simulink model "control_robot"  (R2020a)
settings: Solver=FixedStepAuto  StartTime=0.0  StopTime=inf  FixedStep=0.01  RelTol=1e-3
values from neighbouring files (symbols this model uses):
  alfa = 30*((2*pi)/360)    (= 0.523598775598)    [param.m]
  g = 9.8    [param.m]
  goalLoc = [2 8]    [param.m]
  L = 0.46    [param.m]
  M = 90    [param.m]
  n = 16    [param.m]
  r = 0.125    [param.m]
  simpleMap = [1 1 1 1 1 1 1 1 1 1 1 1 ... (702 elements, 26x27)]    [vid_map.mat]
  startLoc = [2 2]    [param.m]
undefined symbols (not defined in the file or in its folder): DiscIntNeverNeededParam, k_tac, motorIp, motorSp, Pot, sigbuilder_block
libraries: simulink x10, mobileRoboticsTrainingLib x8, robotalgslib x3, commchan3 x2, robotmobilelib x2, robotcorelib x2
settings Model: PacingRate=0.320000  Creator=maxim  LastModifiedBy=maxim

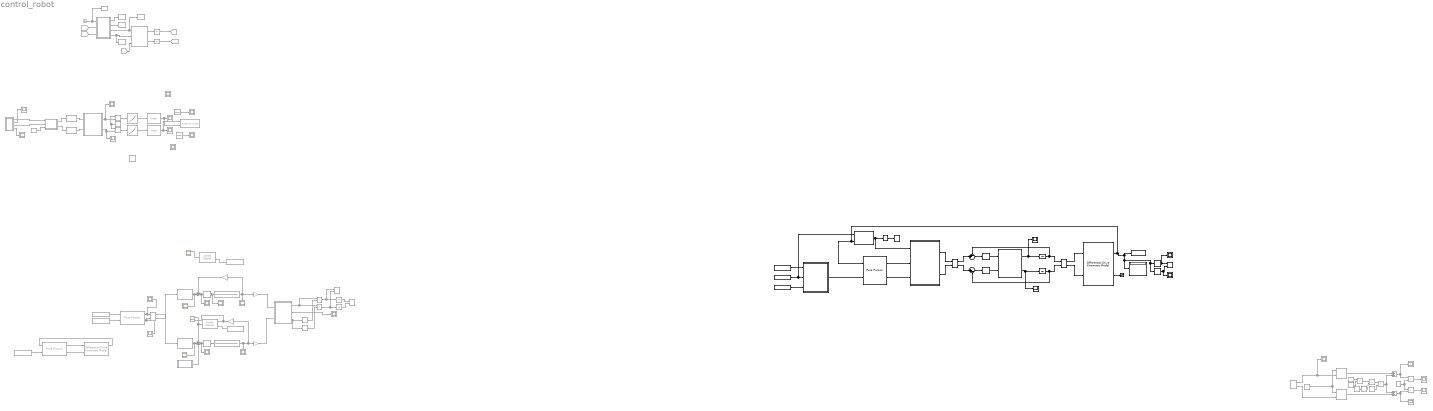
== system control_robot ==
  note: relacion de
      | transmision
  note: Volt_mot = Ktac.Vel_mot
  note: Volt_mot = Ktac.Vel_mot
  note: Voltaje salida
      | motor
  note: rad/s
  note: relacion de
      | transmision
  note: Voltaje salida
      | motor
  note: rad/s
  note: w motor derecho
  note: w motor izquierdo
  note: Robot
  note: Control de Posición
  note: Planificador de Trayectoria
  note: w/T
  note: Control Dinámco
  1-D Lookup Table1 : Lookup_n-D  Commented=on  NumberOfTableDimensions=1  BreakpointsForDimension1=motorSp  Table=motorIp  ExtrapMethod=Clip  InternalRulePriority=Speed  RndMeth=Simplest  InputSameDT=on
  1-D Lookup Table4 : Lookup_n-D  Commented=on  NumberOfTableDimensions=1  BreakpointsForDimension1=motorSp  Table=motorIp  ExtrapMethod=Clip  InternalRulePriority=Speed  RndMeth=Simplest  InputSameDT=on
  AWGN Channel : commchan3/AWGN Channel  Commented=on  InputProcessing=Columns as channels (frame based)  seed=67  noiseMode=Variance from port  EbNodB=10  EsNodB=10  SNRdB=10  bitsPerSym=1  Ps=1  Tsym=1  variance=1
  AWGN Channel1 : commchan3/AWGN Channel  Commented=on  InputProcessing=Columns as channels (frame based)  seed=67  noiseMode=Variance from port  EbNodB=10  EsNodB=10  SNRdB=10  bitsPerSym=1  Ps=1  Tsym=1  variance=1
  Add : Sum  Commented=on
  Add1 : Sum  Commented=on
  Check Distance To Goal : Subsystem
  Cinematica robot diferencial : Subsystem  Commented=on
  Cinematica Inv : robotalgslib/Pure Pursuit  DesiredLinearVelocity=3  MaxAngularVelocity=20  LookaheadDistance=0.5  TargetDirPort=off  SimulateUsing=Code generation
  Cinematica Inversa : Subsystem  Commented=on
  Clock : Clock  Commented=on
      settings: Decimation=40
  Constant : Constant  Commented=on  Value=45
  Constant1 : Constant  Commented=on  Value=Pot
  Constant10 : Constant  Commented=on  Value=alfa
  Constant11 : Constant  Commented=on  Value=r/2
  Constant12 : Constant  Commented=on  Value=1.3
  Constant2 : Constant  Commented=on  Value=[0,0; 5,0; 5,3; 0,3]  VectorParams1D=off  SampleTime=20
  Constant3 : Constant  Commented=on  Value=1570
  Constant4 : Constant  Commented=on  Value=M
  Constant5 : Constant  Commented=on  Value=0.0003  SampleTime=20
  Constant6 : Constant  Commented=on  Value=0.017  SampleTime=20
  Constant7 : Constant  Commented=on  Value=[0,0; 5,0; 5,3; 0,3]  VectorParams1D=off  SampleTime=20
  Constant8 : Constant  Commented=on  Value=[ 0, 0, 0]  SampleTime=20
  Constant9 : Constant  Commented=on  Value=g
  Differential Drive Kinematic Model : robotmobilelib/Differential Drive Kinematic Model  Commented=on  VehicleInputs=Vehicle Speed & Heading Angular Velocity  WheelRadius=r  WheelSpeedRange=[-0.6 0.6]  TrackWidth=0.2  InitialState=[0; 0; 0]  SimulateUsing=Interpreted execution
      settings: SourceProductBaseCode=RO
  Differential Drive Kinematic Model1 : robotmobilelib/Differential Drive Kinematic Model  VehicleInputs=Vehicle Speed & Heading Angular Velocity  WheelRadius=0.05  WheelSpeedRange=[-inf inf]  TrackWidth=0.2  InitialState=[startLoc, 0]'  SimulateUsing=Interpreted execution
      settings: SourceProductBaseCode=RO
  Dinamica Inversa : Subsystem
  Dinamica Inversa2 : Subsystem  Commented=on
  Discrete Derivative : simulink/Discrete/Discrete Derivative  Commented=on  gainval=1.0  ICPrevScaledInput=0.0  OutMin=[]  OutMax=[]  OutDataType=fixdt(1, 16)  OutScaling=2^-10  DoSatur=off
  Discrete Derivative1 : simulink/Discrete/Discrete Derivative  Commented=on  gainval=1.0  ICPrevScaledInput=0.0  OutMin=[]  OutMax=[]  OutDataType=fixdt(1, 16)  OutScaling=2^-10  DoSatur=off
  Discrete-Time Integrator : DiscreteIntegrator  Commented=on  SampleTime=-1  ICPrevOutput=DiscIntNeverNeededParam  ICPrevScaledInput=DiscIntNeverNeededParam
  Discrete-Time Integrator1 : DiscreteIntegrator  Commented=on  SampleTime=-1  ICPrevOutput=DiscIntNeverNeededParam  ICPrevScaledInput=DiscIntNeverNeededParam
  Display : Display
  Divide{,1..3} (4 alike) : Product  Commented=on  Inputs=*/
  From : From  Commented=on  GotoTag=P0
  From1 : From  Commented=on  GotoTag=gamma
  From2 : From  Commented=on  GotoTag=gamma
  Gain1 : Gain  Commented=on  Gain=1/n
  Gain2 : Gain  Commented=on  Gain=k_tac
  Gain4 : Gain  Commented=on  Gain=k_tac
  Gain5 : Gain  Commented=on  Gain=1/n
  Goal Location : Constant  Value=goalLoc
  Goto : Goto  Commented=on  GotoTag=gamma
  Goto1 : Goto  Commented=on  GotoTag=P0
  Integrator : Integrator  Commented=on  InitialCondition=[0;0]
  Integrator1 : Integrator  Commented=on  InitialCondition=[0;0]
  Integrator2 : Integrator  Commented=on
  Integrator3 : Integrator  Commented=on
  MATLAB Function : MATLAB Function  Commented=on  TreatAsAtomicUnit=on
  MATLAB Function1 : MATLAB Function  Commented=on  TreatAsAtomicUnit=on
  Map : Constant  Value=simpleMap
  Motor : mobileRoboticsTrainingLib/Motor  Commented=on  motorPlant=1  sensorType=Position
      settings: SourceProductName=Mobile Robotics Training Library
  Motor Der : TransferFcn  Denominator=[1]
  Motor Izq : TransferFcn  Denominator=[1]
  Motor1 : mobileRoboticsTrainingLib/Motor  Commented=on  motorPlant=1  sensorType=Position
      settings: SourceProductName=Mobile Robotics Training Library
  NOT : Logic  Operator=NOT  IconShape=distinctive  AllPortsSameDT=off  OutDataTypeStr=boolean
  PID Controller : simulink/Continuous/PID Controller  Commented=on  Controller=PID  Form=Parallel  TimeDomain=Discrete-time  UseExternalTs=off  SampleTime=-1  IntegratorMethod=Forward Euler  FilterMethod=Forward Euler  ControllerParametersSource=internal  P=1  I=1  D=0  UseFilter=on  N=100  TunerSelectOption=Transfer Function Based (PID Tuner App)  InitialConditionSource=internal  InitialConditionForIntegrator=0  InitialConditionForFilter=0  DifferentiatorICPrevScaledInput=0  ExternalReset=none  TrackingMode=off  Kt=1  LimitOutput=off  UpperSaturationLimit=inf  LowerSaturationLimit=-inf  LinearizeAsGain=on  AntiWindupMode=none  Kb=1  POutMin=[]  POutMax=[]  IOutMin=[]  IOutMax=[]  DOutMin=[]  DOutMax=[]  NOutMin=[]  NOutMax=[]  SumOutMin=[]  SumOutMax=[]  SaturationOutMin=[]  SaturationOutMax=[]  PParamMin=[]  PParamMax=[]  IParamMin=[]  IParamMax=[]  DParamMin=[]  DParamMax=[]  NParamMin=[]  NParamMax=[]  KbParamMin=[]  KbParamMax=[]  KtParamMin=[]  KtParamMax=[]  KbOutMin=[]  KbOutMax=[]  KtOutMin=[]  KtOutMax=[]  IntegratorOutMin=[]  IntegratorOutMax=[]  FilterOutMin=[]  FilterOutMax=[]  SumI1OutMin=[]  SumI1OutMax=[]  SumI2OutMin=[]  SumI2OutMax=[]  SumI3OutMin=[]  SumI3OutMax=[]  SumI4OutMin=[]  SumI4OutMax=[]  SumDOutMin=[]  SumDOutMax=[]  DifferentiatorOutMin=[]  DifferentiatorOutMax=[]  FilterDiffOutCoefMin=[]  FilterDiffOutCoefMax=[]  ReciprocalOutMin=[]  ReciprocalOutMax=[]  SumDenOutMin=[]  SumDenOutMax=[]  SumNumOutMin=[]  SumNumOutMax=[]  DivideOutMin=[]  DivideOutMax=[]  UdiffTsProdOutMin=[]  UdiffTsProdOutMax=[]  NTsProdOutMin=[]  NTsProdOutMax=[]  UintegralTsProdOutMin=[]  UintegralTsProdOutMax=[]  UngainTsProdOutMin=[]  UngainTsProdOutMax=[]  IntegratorContinuousStateAttributes=''  IntegratorStateMustResolveToSignalObject=off  IntegratorRTWStateStorageClass=Auto  FilterContinuousStateAttributes=''  FilterStateMustResolveToSignalObject=off  FilterRTWStateStorageClass=Auto  ParallelPVariant=InternalParameters  IdealPVariant=Disabled  IVariant=InternalParameters  DVariant=InternalParameters  IntegratorVariant=Discrete  SatVariant=Disabled  AWVariant=Passthrough  PCopyVariant=Disabled  TRVariant=Disabled  FdbkBlocksVariant=Forward  IdealPFdbkVariant=Disabled  SatFdbkVariant=Disabled  DerivativeFilterVariant=ForwardEulerFilter  NVariant=InternalParameters  NCopyVariant=Disabled  FilterICVariant=InternalICsFilter  IntegratorICVariant=InternalICs  ExternalResetVariant=Disabled  TRSumVariant=Passthrough  SumFdbkVariant=Disabled  SumVariant=Sum_PID  TsampFilterVariant=InternalTs  TsampNgainVariant=Passthrough  TsampIntegralVariant=Passthrough  InitialConditionSetting=Output
  PID Controller1 : simulink/Continuous/PID Controller  Commented=on  Controller=PID  Form=Parallel  TimeDomain=Continuous-time  UseExternalTs=off  SampleTime=-1  IntegratorMethod=Forward Euler  FilterMethod=Forward Euler  ControllerParametersSource=internal  P=1.83149033351054  I=8.8184370601147  D=0.0350582199329135  UseFilter=on  N=12.3100428241055  TunerSelectOption=Transfer Function Based (PID Tuner App)  InitialConditionSource=internal  InitialConditionForIntegrator=0  InitialConditionForFilter=0  DifferentiatorICPrevScaledInput=0  ExternalReset=none  TrackingMode=off  Kt=1  LimitOutput=off  UpperSaturationLimit=inf  LowerSaturationLimit=-inf  LinearizeAsGain=on  AntiWindupMode=none  Kb=1  POutMin=[]  POutMax=[]  IOutMin=[]  IOutMax=[]  DOutMin=[]  DOutMax=[]  NOutMin=[]  NOutMax=[]  SumOutMin=[]  SumOutMax=[]  SaturationOutMin=[]  SaturationOutMax=[]  PParamMin=[]  PParamMax=[]  IParamMin=[]  IParamMax=[]  DParamMin=[]  DParamMax=[]  NParamMin=[]  NParamMax=[]  KbParamMin=[]  KbParamMax=[]  KtParamMin=[]  KtParamMax=[]  KbOutMin=[]  KbOutMax=[]  KtOutMin=[]  KtOutMax=[]  IntegratorOutMin=[]  IntegratorOutMax=[]  FilterOutMin=[]  FilterOutMax=[]  SumI1OutMin=[]  SumI1OutMax=[]  SumI2OutMin=[]  SumI2OutMax=[]  SumI3OutMin=[]  SumI3OutMax=[]  SumI4OutMin=[]  SumI4OutMax=[]  SumDOutMin=[]  SumDOutMax=[]  DifferentiatorOutMin=[]  DifferentiatorOutMax=[]  FilterDiffOutCoefMin=[]  FilterDiffOutCoefMax=[]  ReciprocalOutMin=[]  ReciprocalOutMax=[]  SumDenOutMin=[]  SumDenOutMax=[]  SumNumOutMin=[]  SumNumOutMax=[]  DivideOutMin=[]  DivideOutMax=[]  UdiffTsProdOutMin=[]  UdiffTsProdOutMax=[]  NTsProdOutMin=[]  NTsProdOutMax=[]  UintegralTsProdOutMin=[]  UintegralTsProdOutMax=[]  UngainTsProdOutMin=[]  UngainTsProdOutMax=[]  IntegratorContinuousStateAttributes=''  IntegratorStateMustResolveToSignalObject=off  IntegratorRTWStateStorageClass=Auto  FilterContinuousStateAttributes=''  FilterStateMustResolveToSignalObject=off  FilterRTWStateStorageClass=Auto  ParallelPVariant=InternalParameters  IdealPVariant=Disabled  IVariant=InternalParameters  DVariant=InternalParameters  IntegratorVariant=Continuous  SatVariant=Disabled  AWVariant=Passthrough  PCopyVariant=Disabled  TRVariant=Disabled  FdbkBlocksVariant=Forward  IdealPFdbkVariant=Disabled  SatFdbkVariant=Disabled  DerivativeFilterVariant=ContFilter  NVariant=InternalParameters  NCopyVariant=Disabled  FilterICVariant=InternalICsFilter  IntegratorICVariant=InternalICs  ExternalResetVariant=Disabled  TRSumVariant=Passthrough  SumFdbkVariant=Disabled  SumVariant=Sum_PID  TsampFilterVariant=InternalTs  TsampNgainVariant=Passthrough  TsampIntegralVariant=Passthrough
  PID Controller2 : simulink/Continuous/PID Controller  Commented=on  Controller=PID  Form=Parallel  TimeDomain=Continuous-time  UseExternalTs=off  SampleTime=-1  IntegratorMethod=Forward Euler  FilterMethod=Forward Euler  ControllerParametersSource=internal  P=1.83149033351054  I=8.8184370601147  D=0.0350582199329135  UseFilter=on  N=12.3100428241055  TunerSelectOption=Transfer Function Based (PID Tuner App)  InitialConditionSource=internal  InitialConditionForIntegrator=0  InitialConditionForFilter=0  DifferentiatorICPrevScaledInput=0  ExternalReset=none  TrackingMode=off  Kt=1  LimitOutput=off  UpperSaturationLimit=inf  LowerSaturationLimit=-inf  LinearizeAsGain=on  AntiWindupMode=none  Kb=1  POutMin=[]  POutMax=[]  IOutMin=[]  IOutMax=[]  DOutMin=[]  DOutMax=[]  NOutMin=[]  NOutMax=[]  SumOutMin=[]  SumOutMax=[]  SaturationOutMin=[]  SaturationOutMax=[]  PParamMin=[]  PParamMax=[]  IParamMin=[]  IParamMax=[]  DParamMin=[]  DParamMax=[]  NParamMin=[]  NParamMax=[]  KbParamMin=[]  KbParamMax=[]  KtParamMin=[]  KtParamMax=[]  KbOutMin=[]  KbOutMax=[]  KtOutMin=[]  KtOutMax=[]  IntegratorOutMin=[]  IntegratorOutMax=[]  FilterOutMin=[]  FilterOutMax=[]  SumI1OutMin=[]  SumI1OutMax=[]  SumI2OutMin=[]  SumI2OutMax=[]  SumI3OutMin=[]  SumI3OutMax=[]  SumI4OutMin=[]  SumI4OutMax=[]  SumDOutMin=[]  SumDOutMax=[]  DifferentiatorOutMin=[]  DifferentiatorOutMax=[]  FilterDiffOutCoefMin=[]  FilterDiffOutCoefMax=[]  ReciprocalOutMin=[]  ReciprocalOutMax=[]  SumDenOutMin=[]  SumDenOutMax=[]  SumNumOutMin=[]  SumNumOutMax=[]  DivideOutMin=[]  DivideOutMax=[]  UdiffTsProdOutMin=[]  UdiffTsProdOutMax=[]  NTsProdOutMin=[]  NTsProdOutMax=[]  UintegralTsProdOutMin=[]  UintegralTsProdOutMax=[]  UngainTsProdOutMin=[]  UngainTsProdOutMax=[]  IntegratorContinuousStateAttributes=''  IntegratorStateMustResolveToSignalObject=off  IntegratorRTWStateStorageClass=Auto  FilterContinuousStateAttributes=''  FilterStateMustResolveToSignalObject=off  FilterRTWStateStorageClass=Auto  ParallelPVariant=InternalParameters  IdealPVariant=Disabled  IVariant=InternalParameters  DVariant=InternalParameters  IntegratorVariant=Continuous  SatVariant=Disabled  AWVariant=Passthrough  PCopyVariant=Disabled  TRVariant=Disabled  FdbkBlocksVariant=Forward  IdealPFdbkVariant=Disabled  SatFdbkVariant=Disabled  DerivativeFilterVariant=ContFilter  NVariant=InternalParameters  NCopyVariant=Disabled  FilterICVariant=InternalICsFilter  IntegratorICVariant=InternalICs  ExternalResetVariant=Disabled  TRSumVariant=Passthrough  SumFdbkVariant=Disabled  SumVariant=Sum_PID  TsampFilterVariant=InternalTs  TsampNgainVariant=Passthrough  TsampIntegralVariant=Passthrough
  PID Controller3 : simulink/Continuous/PID Controller  Controller=PID  Form=Parallel  TimeDomain=Continuous-time  UseExternalTs=off  SampleTime=-1  IntegratorMethod=Forward Euler  FilterMethod=Forward Euler  ControllerParametersSource=internal  P=0  I=0  D=0  UseFilter=on  N=100  TunerSelectOption=Transfer Function Based (PID Tuner App)  InitialConditionSource=internal  InitialConditionForIntegrator=0  InitialConditionForFilter=0  DifferentiatorICPrevScaledInput=0  ExternalReset=none  TrackingMode=off  Kt=1  LimitOutput=off  UpperSaturationLimit=inf  LowerSaturationLimit=-inf  LinearizeAsGain=on  AntiWindupMode=none  Kb=1  POutMin=[]  POutMax=[]  IOutMin=[]  IOutMax=[]  DOutMin=[]  DOutMax=[]  NOutMin=[]  NOutMax=[]  SumOutMin=[]  SumOutMax=[]  SaturationOutMin=[]  SaturationOutMax=[]  PParamMin=[]  PParamMax=[]  IParamMin=[]  IParamMax=[]  DParamMin=[]  DParamMax=[]  NParamMin=[]  NParamMax=[]  KbParamMin=[]  KbParamMax=[]  KtParamMin=[]  KtParamMax=[]  KbOutMin=[]  KbOutMax=[]  KtOutMin=[]  KtOutMax=[]  IntegratorOutMin=[]  IntegratorOutMax=[]  FilterOutMin=[]  FilterOutMax=[]  SumI1OutMin=[]  SumI1OutMax=[]  SumI2OutMin=[]  SumI2OutMax=[]  SumI3OutMin=[]  SumI3OutMax=[]  SumI4OutMin=[]  SumI4OutMax=[]  SumDOutMin=[]  SumDOutMax=[]  DifferentiatorOutMin=[]  DifferentiatorOutMax=[]  FilterDiffOutCoefMin=[]  FilterDiffOutCoefMax=[]  ReciprocalOutMin=[]  ReciprocalOutMax=[]  SumDenOutMin=[]  SumDenOutMax=[]  SumNumOutMin=[]  SumNumOutMax=[]  DivideOutMin=[]  DivideOutMax=[]  UdiffTsProdOutMin=[]  UdiffTsProdOutMax=[]  NTsProdOutMin=[]  NTsProdOutMax=[]  UintegralTsProdOutMin=[]  UintegralTsProdOutMax=[]  UngainTsProdOutMin=[]  UngainTsProdOutMax=[]  IntegratorContinuousStateAttributes=''  IntegratorStateMustResolveToSignalObject=off  IntegratorRTWStateStorageClass=Auto  FilterContinuousStateAttributes=''  FilterStateMustResolveToSignalObject=off  FilterRTWStateStorageClass=Auto  ParallelPVariant=InternalParameters  IdealPVariant=Disabled  IVariant=InternalParameters  DVariant=InternalParameters  IntegratorVariant=Continuous  SatVariant=Disabled  AWVariant=Passthrough  PCopyVariant=Disabled  TRVariant=Disabled  FdbkBlocksVariant=Forward  IdealPFdbkVariant=Disabled  SatFdbkVariant=Disabled  DerivativeFilterVariant=ContFilter  NVariant=InternalParameters  NCopyVariant=Disabled  FilterICVariant=InternalICsFilter  IntegratorICVariant=InternalICs  ExternalResetVariant=Disabled  TRSumVariant=Passthrough  SumFdbkVariant=Disabled  SumVariant=Sum_PID  TsampFilterVariant=InternalTs  TsampNgainVariant=Passthrough  TsampIntegralVariant=Passthrough
  PID Controller4 : simulink/Continuous/PID Controller  Controller=PID  Form=Parallel  TimeDomain=Continuous-time  UseExternalTs=off  SampleTime=-1  IntegratorMethod=Forward Euler  FilterMethod=Forward Euler  ControllerParametersSource=internal  P=0  I=0  D=0  UseFilter=on  N=100  TunerSelectOption=Transfer Function Based (PID Tuner App)  InitialConditionSource=internal  InitialConditionForIntegrator=0  InitialConditionForFilter=0  DifferentiatorICPrevScaledInput=0  ExternalReset=none  TrackingMode=off  Kt=1  LimitOutput=off  UpperSaturationLimit=inf  LowerSaturationLimit=-inf  LinearizeAsGain=on  AntiWindupMode=none  Kb=1  POutMin=[]  POutMax=[]  IOutMin=[]  IOutMax=[]  DOutMin=[]  DOutMax=[]  NOutMin=[]  NOutMax=[]  SumOutMin=[]  SumOutMax=[]  SaturationOutMin=[]  SaturationOutMax=[]  PParamMin=[]  PParamMax=[]  IParamMin=[]  IParamMax=[]  DParamMin=[]  DParamMax=[]  NParamMin=[]  NParamMax=[]  KbParamMin=[]  KbParamMax=[]  KtParamMin=[]  KtParamMax=[]  KbOutMin=[]  KbOutMax=[]  KtOutMin=[]  KtOutMax=[]  IntegratorOutMin=[]  IntegratorOutMax=[]  FilterOutMin=[]  FilterOutMax=[]  SumI1OutMin=[]  SumI1OutMax=[]  SumI2OutMin=[]  SumI2OutMax=[]  SumI3OutMin=[]  SumI3OutMax=[]  SumI4OutMin=[]  SumI4OutMax=[]  SumDOutMin=[]  SumDOutMax=[]  DifferentiatorOutMin=[]  DifferentiatorOutMax=[]  FilterDiffOutCoefMin=[]  FilterDiffOutCoefMax=[]  ReciprocalOutMin=[]  ReciprocalOutMax=[]  SumDenOutMin=[]  SumDenOutMax=[]  SumNumOutMin=[]  SumNumOutMax=[]  DivideOutMin=[]  DivideOutMax=[]  UdiffTsProdOutMin=[]  UdiffTsProdOutMax=[]  NTsProdOutMin=[]  NTsProdOutMax=[]  UintegralTsProdOutMin=[]  UintegralTsProdOutMax=[]  UngainTsProdOutMin=[]  UngainTsProdOutMax=[]  IntegratorContinuousStateAttributes=''  IntegratorStateMustResolveToSignalObject=off  IntegratorRTWStateStorageClass=Auto  FilterContinuousStateAttributes=''  FilterStateMustResolveToSignalObject=off  FilterRTWStateStorageClass=Auto  ParallelPVariant=InternalParameters  IdealPVariant=Disabled  IVariant=InternalParameters  DVariant=InternalParameters  IntegratorVariant=Continuous  SatVariant=Disabled  AWVariant=Passthrough  PCopyVariant=Disabled  TRVariant=Disabled  FdbkBlocksVariant=Forward  IdealPFdbkVariant=Disabled  SatFdbkVariant=Disabled  DerivativeFilterVariant=ContFilter  NVariant=InternalParameters  NCopyVariant=Disabled  FilterICVariant=InternalICsFilter  IntegratorICVariant=InternalICs  ExternalResetVariant=Disabled  TRSumVariant=Passthrough  SumFdbkVariant=Disabled  SumVariant=Sum_PID  TsampFilterVariant=InternalTs  TsampNgainVariant=Passthrough  TsampIntegralVariant=Passthrough
  Planner : MATLAB Function  TreatAsAtomicUnit=on
  Product{,1..6} (7 alike) : Product  Commented=on
  Pure Pursuit : robotalgslib/Pure Pursuit  Commented=on  DesiredLinearVelocity=3  MaxAngularVelocity=20  LookaheadDistance=0.5  TargetDirPort=off  SimulateUsing=Interpreted execution
  Pure Pursuit1 : robotalgslib/Pure Pursuit  Commented=on  DesiredLinearVelocity=3  MaxAngularVelocity=20  LookaheadDistance=0.5  TargetDirPort=off  SimulateUsing=Interpreted execution
  Px vs Py : simulink/Sinks/XY Graph  Commented=on  xmin=-5  xmax=5  ymin=-5  ymax=5  st=-1
  Robot Simulator1 : mobileRoboticsTrainingLib/Robot Simulator  Priority=99  Commented=on  mapVar=[]  startX=1  startY=1  startTheta=0  axleLength=0.1  wheelR=0.05
  Scope{,1..13,15..17,19..21} (20 alike) : Scope  Commented=on
  Scope14 : Scope  Commented=on  NumInputPorts=2
  Scope18 : Scope  Commented=on  NumInputPorts=2
  Selector : Selector  InputPortWidth=3  IndexOptions=Index vector (dialog)  Indices=[1]  OutputSizes=1
  Selector1 : Selector  InputPortWidth=3  IndexOptions=Index vector (dialog)  Indices=[2]  OutputSizes=1
  Signal Builder : Subsystem  Tag=STV Subsys  Commented=on  LoadFcn=sigbuilder_block('load');  StartFcn=sigbuilder_block('start');  StopFcn=sigbuilder_block('stop');  ClipboardFcn=sigbuilder_block('clipboard');  mask(Sigbuilder block){tuvar=[0:10]}
      mask help: Simulink:masks:SigbuilderBlock_MD
      mask init:
      | if ~strcmp(get_param(bdroot(gcbh),'SimulationStatus'),'stopped') tuvar = sigbuilder_block('maskInit'); end
      settings: CopyFcn=sigbuilder_block('copy');  DeleteFcn=sigbuilder_block('delete');  ModelCloseFcn=sigbuilder_block('modelClose');  PreSaveFcn=sigbuilder_block('preSave');  PauseFcn=sigbuilder_block('pause');  ContinueFcn=sigbuilder_block('continue');  NameChangeFcn=sigbuilder_block('namechange');  OpenFcn=sigbuilder_block('open',[321 79.8 550.8 400.2 ]);  CloseFcn=sigbuilder_block('close');
      mask Display: plot(0, 0, 100, 100,[2, 2, 32, 32, 2], [68, 8, 8, 68, 68],[32, 2], [38, 38], [32, 19, 2],[53, 60, 44], [32, 17, 17, 2],[16, 16, 31, 31]);txt = getActiveGroup(gcbh);text(2, 100, txt,'verticalAlignment', 'top');
  Sin : Trigonometry  Commented=on
  Start Location : Constant  Value=startLoc
  Stop Simulation : Stop
  Sum : Sum  Commented=on  Inputs=-+|
  Sum1 : Sum  Inputs=-+|
  Sum2 : Sum  Commented=on  Inputs=-+-
  Sum3 : Sum  Inputs=|+-
  Terminator : Terminator
  To Workspace : ToWorkspace  VariableName=Pose  SampleTime=-1
  To Workspace1 : ToWorkspace  Commented=on  VariableName=v  SampleTime=-1
  To Workspace2 : ToWorkspace  Commented=on  VariableName=t  SampleTime=-1
  To Workspace3 : ToWorkspace  Commented=on  VariableName=P  SampleTime=-1
  To Workspace4 : ToWorkspace  Commented=on  VariableName=Pd  SampleTime=-1
  To Workspace5 : ToWorkspace  Commented=on  VariableName=w  SampleTime=-1
  To vw : mobileRoboticsTrainingLib/To vw  axleLength=0.1  wheelR=0.05
      settings: SourceProductName=Mobile Robotics Training Library
  To wlwr : mobileRoboticsTrainingLib/To wlwr  Commented=on  axleLength=L  wheelR=r
      link override change parameters: Gain=[1 -L/2; 1 L/2]
      link override vtow: Gain=1/r
  To wlwr1 : mobileRoboticsTrainingLib/To wlwr  axleLength=0.1  wheelR=0.05
  To wlwr3 : mobileRoboticsTrainingLib/To wlwr  Commented=on  axleLength=0.1  wheelR=0.05
  Torque Der1 : Scope  Commented=on
  Torque Der2 : Scope  Commented=on
  Torque Derecho : Scope
  Torque Izq1 : Scope  Commented=on
  Torque Izq2 : Scope  Commented=on
  Torque Izq6 : Scope  Commented=on
  Torque Izquierdo : Scope
  Trayectoria : Subsystem  Commented=on
  Trigonometric Function : Trigonometry  Commented=on
  Trigonometric Function1 : Trigonometry  Commented=on  Operator=cos
  Vx vs Vy : simulink/Sinks/XY Graph  Commented=on  xmin=-0.2  xmax=0.2  ymin=-0.2  ymax=0.2  st=-1
  XY Graph : simulink/Sinks/XY Graph  xmin=0  xmax=28  ymin=0  ymax=28  st=-1
  Zero-Velocity At Goal : Subsystem
  vel angular motor / voltaje : TransferFcn  Commented=on  Numerator=[0.112]  Denominator=[5.3e-5 0.031 0.109]
  vel angular motor / voltaje1 : TransferFcn  Commented=on  Numerator=[0.062]  Denominator=[5.3e-5 0.031 0.109]
  vel2volt : Subsystem  Commented=on
  vel2volt1 : Subsystem  Commented=on
  x : Scope
  y : Scope
  wires:
  Clock/1 -> To Workspace2/1, MATLAB Function/1(t)
  MATLAB Function/3(v) -> To Workspace1/1, MATLAB Function1/1(v)
  From1/1 -> MATLAB Function/3(gamma)
  From/1 -> MATLAB Function/2(P0)
  MATLAB Function/2(P) -> To Workspace3/1
  MATLAB Function/1(Pd) -> To Workspace4/1
  MATLAB Function/4(w) -> To Workspace5/1, MATLAB Function1/2(w)
  MATLAB Function1/1(dP0) -> Integrator/1
  MATLAB Function1/2(dgamma) -> Integrator1/1
  Integrator1/1 -> Goto/1
  Integrator/1 -> Goto1/1
  From2/1 -> MATLAB Function1/3(gamma)
  Discrete-Time Integrator/1 -> Scope2/1
  Discrete-Time Integrator1/1 -> Scope3/1
  Cinematica Inversa/2(wl) -> Discrete Derivative/1
  Discrete Derivative/1 -> Dinamica Inversa2/2(ddthetaL)
  Cinematica Inversa/1(wr) -> Discrete Derivative1/1
  Discrete Derivative1/1 -> Dinamica Inversa2/1(ddthetaR)
  Dinamica Inversa2/2(tauTot_L) -> Divide1/2, Scope5/1
  Trayectoria/1(x) -> Cinematica Inversa/1(xd)
  Trayectoria/3(y) -> Cinematica Inversa/2(yd)
  Trayectoria/2(dx) -> Scope6/1
  Trayectoria/4(dy) -> Scope7/1
  Constant/1 -> Cinematica Inversa/3(gamma)
  Dinamica Inversa2/1(tauTot_R) -> Divide/2, Scope4/1
  Constant1/1 -> Divide1/1, Divide/1
  Divide/1 -> 1-D Lookup Table4/1
  1-D Lookup Table1/1 -> Motor1/1
  1-D Lookup Table4/1 -> Motor/1
  Divide1/1 -> 1-D Lookup Table1/1
  Motor/1 -> Robot Simulator1/2, Scope8/1
  Motor1/1 -> Robot Simulator1/1, Scope9/1
  vel angular motor / voltaje/1 -> Gain2/1, Scope10/1, Gain1/1
  Gain5/1 -> Cinematica robot diferencial/2(w_l)
  Trigonometric Function/1 -> Product/2
  Constant8/1 -> Pure Pursuit/1
  PID Controller1/1 -> Scope11/1, vel angular motor / voltaje/1
  Product/1 -> Integrator2/1, Vx vs Vy/1
  Pure Pursuit/2 -> Scope21/1, To wlwr/2
  Constant6/1 -> AWGN Channel1/2
  Cinematica robot diferencial/1(v robot) -> Product/1, Product1/1
  To wlwr/2 -> vel2volt/1(vel motor)
  Cinematica robot diferencial/2(w robot) -> Scope15/1
  Integrator3/1 -> Px vs Py/2
  AWGN Channel1/1 -> Scope14/1, Sum2/1
  To wlwr/1 -> vel2volt1/1(vel motor)
  PID Controller2/1 -> vel angular motor / voltaje1/1
  Signal Builder/1(Pert) -> Sum2/3
  Trigonometric Function1/1 -> Product1/2
  Gain1/1 -> Cinematica robot diferencial/1(w_r)
  vel angular motor / voltaje1/1 -> Gain5/1, Gain4/1, Scope19/1
  Cinematica robot diferencial/3(theta) -> Trigonometric Function1/1, Trigonometric Function/1
  Gain4/1 -> Scope14/2, AWGN Channel1/1
  Pure Pursuit/1 -> Scope20/1, To wlwr/1
  Constant5/1 -> AWGN Channel/2
  Sum/1 -> Scope16/1, PID Controller1/1
  Constant7/1 -> Pure Pursuit/2
  Sum2/1 -> PID Controller2/1, Scope12/1
  AWGN Channel/1 -> Scope18/1
  Product1/1 -> Vx vs Vy/2, Integrator3/1
  Integrator2/1 -> Px vs Py/1
  vel2volt/1(voltaje) -> Scope17/1, Sum/2
  vel2volt1/1(voltaje) -> Sum2/2, Scope13/1
  Gain2/1 -> Sum/1
  Pure Pursuit1/1 -> Differential Drive Kinematic Model/1
  Pure Pursuit1/2 -> Differential Drive Kinematic Model/2
  Constant2/1 -> Pure Pursuit1/2
  Differential Drive Kinematic Model/1 -> Pure Pursuit1/1
  Map/1 -> Planner/3(mapMatrix)
  Differential Drive Kinematic Model1/2 -> Terminator/1
  NOT/1 -> Stop Simulation/1
  Differential Drive Kinematic Model1/1 -> To Workspace/1, Selector1/1, Selector/1, Display/1, Cinematica Inv/1, Check Distance To Goal/2(currentPose)
  Start Location/1 -> Planner/1(startPos)
  Cinematica Inv/1 -> Zero-Velocity At Goal/2(linearVelocityOutput)  "linearVelocityOutput"
  Selector1/1 -> y/1, XY Graph/2
  Check Distance To Goal/1(atGoal) -> Zero-Velocity At Goal/1(atGoal), NOT/1
  Cinematica Inv/2 -> Zero-Velocity At Goal/3(angularVelocityOutput)  "angularVelocityOutput"
  Planner/1(waypoints) -> Cinematica Inv/2  "planOutput"
  Goal Location/1 -> Check Distance To Goal/1(robotGoal), Planner/2(endPos)
  Product5/1 -> Torque Izq2/1
  Product6/1 -> Torque Der2/1
  Constant3/1 -> Divide2/1, Divide3/1
  Selector/1 -> x/1, XY Graph/1
  Constant4/1 -> Product2/1
  Constant9/1 -> Product2/2
  Product2/1 -> Product3/1
  Constant10/1 -> Sin/1
  Sin/1 -> Product3/2
  Add/1 -> Torque Izq1/1, Product5/1
  Divide2/1 -> Add/1
  Add1/1 -> Product6/2, Torque Der1/1
  Divide3/1 -> Add1/2
  Product3/1 -> Product4/1
  Constant11/1 -> Product4/2
  Product4/1 -> Add/2, Add1/1
  Constant12/1 -> Product6/1, Product5/2
  Dinamica Inversa/2(tauTot_R) -> Motor Der/1, Torque Derecho/1
  Dinamica Inversa/1(tauTot_L) -> Motor Izq/1, Torque Izquierdo/1
  To wlwr3/1 -> Torque Izq6/1, Divide2/2
  To wlwr3/2 -> Divide3/2
  Sum1/1 -> PID Controller3/1
  Sum3/1 -> PID Controller4/1
  Motor Der/1 -> To vw/2, Sum3/2
  Motor Izq/1 -> To vw/1, Sum1/1
  To vw/1 -> Differential Drive Kinematic Model1/1
  To vw/2 -> Differential Drive Kinematic Model1/2
  To wlwr1/1 -> Sum1/2
  To wlwr1/2 -> Sum3/1
  PID Controller3/1 -> Dinamica Inversa/1(ddthetaR)
  PID Controller4/1 -> Dinamica Inversa/2(ddthetaL)
  Zero-Velocity At Goal/1(Linear Velocity) -> To wlwr1/1
  Zero-Velocity At Goal/2(Angular Velocity) -> To wlwr1/2

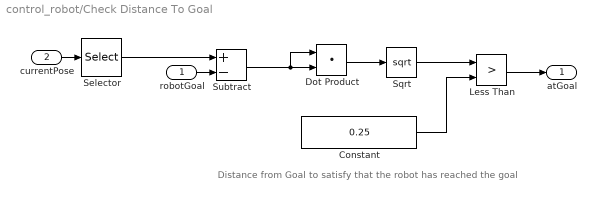
== system control_robot/Check Distance To Goal ==
  note: Distance from Goal to satisfy that the robot has reached the goal
  robotGoal : Inport
  currentPose : Inport  Port=2
  Constant : Constant  Value=0.25
  Dot Product : DotProduct  InputSameDT=on  OutDataTypeStr=Inherit: Inherit via internal rule
  Less Than : RelationalOperator  Operator=>  OutDataTypeStr=boolean  RndMeth=Simplest
  Selector : Selector  InputPortWidth=3  IndexOptions=Index vector (dialog)  Indices=[1 2]  OutputSizes=1
  Sqrt : Sqrt  SaturateOnIntegerOverflow=on
  Subtract : Sum  Inputs=+-
  atGoal : Outport
  wires:
  robotGoal/1 -> Subtract/2
  Dot Product/1 -> Sqrt/1
  Constant/1 -> Less Than/2
  currentPose/1 -> Selector/1
  Less Than/1 -> atGoal/1
  Sqrt/1 -> Less Than/1
  Subtract/1 -> Dot Product/1, Dot Product/2
  Selector/1 -> Subtract/1

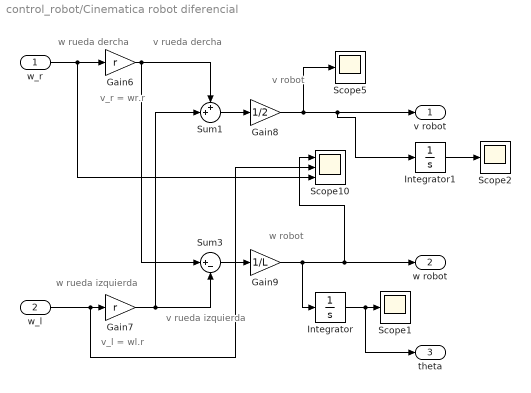
== system control_robot/Cinematica robot diferencial ==
  note: w rueda
      | dercha
  note: w rueda
      | izquierda
  note: v_r = wr.r
  note: v_l = wl.r
  note: v robot
  note: w robot
  note: v rueda
      | dercha
  note: v rueda
      | izquierda
  w_r : Inport
  w_l : Inport  Port=2
  Gain6 : Gain  Gain=r
  Gain7 : Gain  Gain=r
  Gain8 : Gain  Gain=1/2
  Gain9 : Gain  Gain=1/L
  Integrator : Integrator
  Integrator1 : Integrator
  Scope1 : Scope
  Scope10 : Scope  NumInputPorts=3
  Scope2 : Scope
  Scope5 : Scope
  Sum1 : Sum  Inputs=++|
  Sum3 : Sum  Inputs=|+-
  v robot : Outport
  w robot : Outport  Port=2
  theta : Outport  Port=3
  wires:
  w_l/1 -> Scope10/2, Gain7/1
  Sum3/1 -> Gain9/1
  Gain9/1 -> Integrator/1, w robot/1, Scope10/1
  Gain7/1 -> Sum3/2, Sum1/2
  Gain6/1 -> Sum3/1, Sum1/1
  Sum1/1 -> Gain8/1
  w_r/1 -> Scope10/3, Gain6/1
  Gain8/1 -> Scope5/1, Integrator1/1, v robot/1
  Integrator/1 -> theta/1, Scope1/1
  Integrator1/1 -> Scope2/1

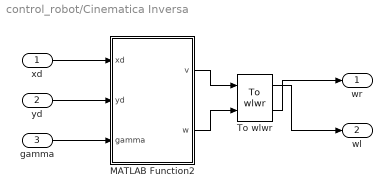
== system control_robot/Cinematica Inversa ==
  xd : Inport
  yd : Inport  Port=2
  gamma : Inport  Port=3
  MATLAB Function2 : MATLAB Function  TreatAsAtomicUnit=on
  To wlwr : mobileRoboticsTrainingLib/To wlwr  axleLength=L  wheelR=r
      link override change parameters: Gain=[1 -L/2; 1 L/2]
      link override vtow: Gain=1/r
  wr : Outport
  wl : Outport  Port=2
  wires:
  MATLAB Function2/2(w) -> To wlwr/2
  MATLAB Function2/1(v) -> To wlwr/1
  gamma/1 -> MATLAB Function2/3(gamma)
  yd/1 -> MATLAB Function2/2(yd)
  xd/1 -> MATLAB Function2/1(xd)
  To wlwr/2 -> wr/1
  To wlwr/1 -> wl/1

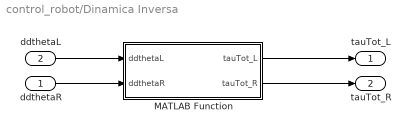
== system control_robot/Dinamica Inversa ==
  ddthetaR : Inport
  ddthetaL : Inport  Port=2
  MATLAB Function : MATLAB Function  TreatAsAtomicUnit=on
  tauTot_L : Outport
  tauTot_R : Outport  Port=2
  wires:
  ddthetaL/1 -> MATLAB Function/1(ddthetaL)
  ddthetaR/1 -> MATLAB Function/2(ddthetaR)
  MATLAB Function/2(tauTot_R) -> tauTot_R/1
  MATLAB Function/1(tauTot_L) -> tauTot_L/1

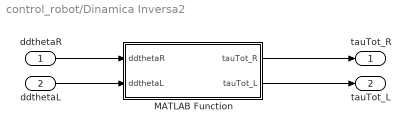
== system control_robot/Dinamica Inversa2 ==
  ddthetaR : Inport
  ddthetaL : Inport  Port=2
  MATLAB Function : MATLAB Function  TreatAsAtomicUnit=on
  tauTot_R : Outport
  tauTot_L : Outport  Port=2
  wires:
  ddthetaL/1 -> MATLAB Function/2(ddthetaL)
  ddthetaR/1 -> MATLAB Function/1(ddthetaR)
  MATLAB Function/1(tauTot_R) -> tauTot_R/1
  MATLAB Function/2(tauTot_L) -> tauTot_L/1

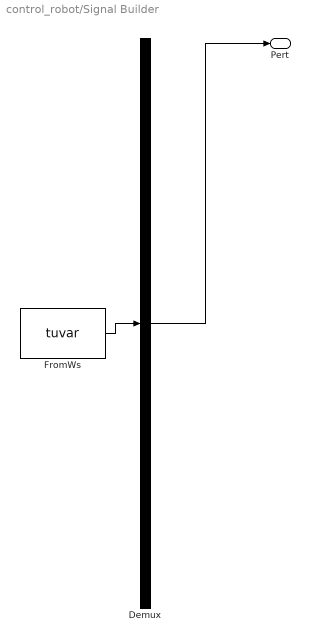
== system control_robot/Signal Builder ==
  Demux : Demux  Tag=STV Demux  Outputs=1
      settings: DisplayOption=none
  FromWs : FromWorkspace  Tag=STV FromWs  VariableName=tuvar  SampleTime=0.01
      SigBuilderData=|
      | common.afterFinalStr = 'Extrapolate'
      | common.sampleTime = '0.01'
      | dataSet.timeRange = [0 20]
      | dataSet.name = 'Group 1'
      | sbobj.Groups.Name = 'Group 1'
      | sbobj.Groups.Signals.Name = 'Pert'
      | sbobj.Groups.Signals.XData = [0 4 4 6 6 20]
      | sbobj.Groups.Signals.YData = [0 0 1 1 0 0]
      | sbobj.Groups.TimeRange = [0 20]
  Pert : Outport  Tag=STV Outport
  wires:
  Demux/1 -> Pert/1
  FromWs/1 -> Demux/1

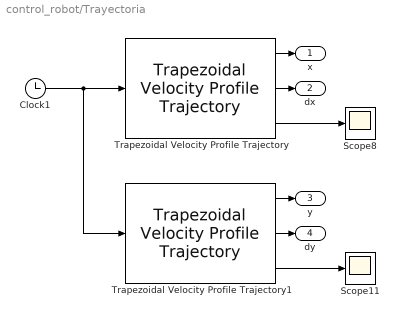
== system control_robot/Trayectoria ==
  Clock1 : Clock
  Scope11 : Scope
  Scope8 : Scope
  Trapezoidal Velocity Profile Trajectory : robotcorelib/Trapezoidal Velocity Profile Trajectory  WaypointSource=Internal  Waypoints=[ 0, -0.5, -1 ]  NumParams=0  Parameter1=Peak Velocity  Parameter2=End Time  ParameterSource=Internal  PeakVelocity=[ 2; 2 ]  Acceleration=[ 1; 2 ]  EndTime=[ 1; 1 ]  AccelTime=[ 1; 2 ]  SimulateUsing=Interpreted execution
      settings: SourceProductBaseCode=NV,RO,RR
  Trapezoidal Velocity Profile Trajectory1 : robotcorelib/Trapezoidal Velocity Profile Trajectory  WaypointSource=Internal  Waypoints=[ 0, 0.5, 1 ]  NumParams=0  Parameter1=Peak Velocity  Parameter2=End Time  ParameterSource=Internal  PeakVelocity=[ 2; 2 ]  Acceleration=[ 1; 2 ]  EndTime=[ 1; 1 ]  AccelTime=[ 1; 2 ]  SimulateUsing=Interpreted execution
      settings: SourceProductBaseCode=NV,RO,RR
  x : Outport
  dx : Outport  Port=2
  y : Outport  Port=3
  dy : Outport  Port=4
  wires:
  Trapezoidal Velocity Profile Trajectory1/3 -> Scope11/1
  Trapezoidal Velocity Profile Trajectory/3 -> Scope8/1
  Trapezoidal Velocity Profile Trajectory1/1 -> y/1
  Trapezoidal Velocity Profile Trajectory/2 -> dx/1
  Clock1/1 -> Trapezoidal Velocity Profile Trajectory1/1, Trapezoidal Velocity Profile Trajectory/1
  Trapezoidal Velocity Profile Trajectory1/2 -> dy/1
  Trapezoidal Velocity Profile Trajectory/1 -> x/1

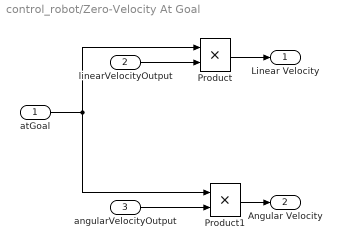
== system control_robot/Zero-Velocity At Goal ==
  atGoal : Inport
  linearVelocityOutput : Inport  Port=2
  angularVelocityOutput : Inport  Port=3
  Product : Product
  Product1 : Product
  Linear Velocity : Outport  OutDataTypeStr=double
  Angular Velocity : Outport  Port=2  OutDataTypeStr=double
  wires:
  atGoal/1 -> Product1/1, Product/1
  angularVelocityOutput/1 -> Product1/2
  linearVelocityOutput/1 -> Product/2
  Product/1 -> Linear Velocity/1
  Product1/1 -> Angular Velocity/1

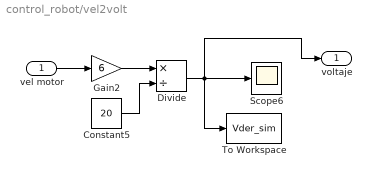
== system control_robot/vel2volt ==
  vel motor : Inport
  Constant5 : Constant  Value=20
  Divide : Product  Inputs=*/
  Gain2 : Gain  Gain=6
  Scope6 : Scope
  To Workspace : ToWorkspace  VariableName=Vder_sim  SampleTime=-1
  voltaje : Outport
  wires:
  Divide/1 -> voltaje/1, Scope6/1, To Workspace/1
  Gain2/1 -> Divide/1
  Constant5/1 -> Divide/2
  vel motor/1 -> Gain2/1

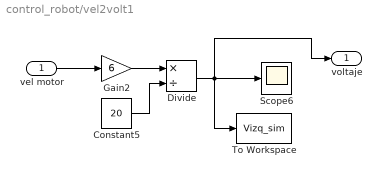
== system control_robot/vel2volt1 ==
  vel motor : Inport
  Constant5 : Constant  Value=20
  Divide : Product  Inputs=*/
  Gain2 : Gain  Gain=6
  Scope6 : Scope
  To Workspace : ToWorkspace  VariableName=Vizq_sim  SampleTime=-1
  voltaje : Outport
  wires:
  vel motor/1 -> Gain2/1
  Constant5/1 -> Divide/2
  Gain2/1 -> Divide/1
  Divide/1 -> To Workspace/1, Scope6/1, voltaje/1

== matlab function control_robot/MATLAB Function1 ==
  data: v input; w input; gamma input; dP0 output; dgamma output
function [dP0,dgamma] = SNL(v, w, gamma)
dP0 = [v*cos(gamma); v*sin(gamma)]
dgamma = w;

== matlab function control_robot/MATLAB Function ==
  data: Pd output; P output; t input; P0 input; v output; gamma input; w output
function [Pd, P, v, w] = Pout(t, P0, gamma)
%control tomando un punto por fuera
d = 0.1; kp = 2;

%trayectoria deseada
T=40;
b = 2*pi/T;
Pd = [cos(b*t); sin(b*t)];
dPd = [-b*sin(b*t); b*cos(b*t)];

%Punto por fuera del eje de las ruedas
P = [P0(1)+d*cos(gamma); P0(2)+d*sin(gamma)];

%Error de seguimiento
e = Pd-P;

%Matriz de desacoplamiento o Jacboiano
A = [cos(gamma), -d*sin(gamma);
     sin(gamma), d*cos(gamma)];

 %Control P con compensación
 u = dPd + kp*e;
 U = A\u;
 v = U(1);
 w = U(2);

== matlab function control_robot/Cinematica Inversa/MATLAB Function2 ==
  data: xd input; yd input; v output; gamma input; w output
 function [v, w] = cin_inv(xd, yd, gamma)
%control tomando un punto por fuera
a = 0.445; 

%Matriz de desacoplamiento o Jacboiano
A = [cos(gamma), -a*sin(gamma);
     sin(gamma), a*cos(gamma)]

%Control P con compensación
P = [xd; yd];
U = A^(-1)*P ;
v = U(1);
w = U(2);

== matlab function control_robot/Dinamica Inversa2/MATLAB Function ==
  data: ddthetaR input; ddthetaL input; tauTot_R output; tauTot_L output
function [tauTot_R, tauTot_L] = din_inv(ddthetaR, ddthetaL)

a = 0.445;
L = 0.46;
r = 0.125;

M = 90;
mg = 1.5;
mc = 1;
rc = 0.08;
I = 8.53;
alfa = 30;
mu = 80;
g = 9.8;


ddtheta = [ddthetaR; ddthetaL] %Vector de aceleraciones
D = (r/(L^2))*[(M*(a^2) + 1/4 + I +(M*a*L)/r + 2*(L^2)*(2*mc + mg)),  -(M*(a^2) + 1/4 - I);
                  -(M*(a^2) + 1/4 - I), (M*(a^2) + 1/4 + I -(M*a*L)/r + 2*(L^2)*(2*mc + mg))]; %Matriz de inercia

tau_ef = D * ddtheta;

tau_fric = 0.3 * tau_ef; %Torques de friccion

tau_pend = (r/2)*mu*g*sin(alfa)*[1;1]; %Torques de pendiente de 30 grados

tauTot = tau_ef + tau_fric + tau_pend;

tauTot_R = tauTot(1); 
tauTot_L = tauTot(2);

== matlab function control_robot/Planner ==
  settings: updateMethod=DISCRETE
  data: startPos input size=[1 2]; endPos input size=[1 2]; waypoints output size=[100 2]; mapMatrix input
function waypoints = planning(startPos, endPos, mapMatrix)

persistent waypointsInternal
persistent prevStartPos
persistent prevEndPos

% Set constant parameters
maxNumNodes = 100;

% Initialize persistent variables that are used downstream
if isempty(prevStartPos)
    prevStartPos = startPos;
end

if isempty(prevEndPos)
    prevEndPos = endPos;
end

isNewPath = (~isequal(prevStartPos, startPos) || ~isequal(prevEndPos, endPos));

if isempty(waypointsInternal) || isNewPath
    % Two conditions in which waypoints must be set: they are not yet
    % initialized, or they are initialized, but the current start and end
    % do not match those used to generate the previous set of waypoints
    [waypointsInternal] = planPath(mapMatrix, maxNumNodes, startPos, endPos);
end

% Update the outputs
waypoints = waypointsInternal;

% Update the persistent variables that indicate previous state
prevStartPos = startPos;
prevEndPos = endPos;

%% Helper Function

function wayPoints = planPath(mapMatrix, maxNodes, startPos, endPos)
    
    % Create a probabilistic roadmap
    map = binaryOccupancyMap(mapMatrix);
    prm = mobileRobotPRM(map, maxNodes);
    
    % Find a path between two points
    xy = findpath(prm, startPos, endPos);
    wayPoints = repmat(endPos, maxNodes, 1);
    
    % Number of nodes that are actually used
    numNodes = length(xy);
    wayPoints(1:numNodes,:) = xy;    

end

end

== matlab function control_robot/Dinamica Inversa/MATLAB Function ==
  data: ddthetaL input; tauTot_L output; ddthetaR input; tauTot_R output
function [tauTot_L, tauTot_R] = din_inv(ddthetaL, ddthetaR)

a=0.445;
L=0.46;
r=0.125;
M=90;
mg=1.5;
mc=1;
rc=0.08;
P=1570;
I=8.53;
alfa=30*((2*pi)/360);
mu=80;
g=9.8;


ddtheta = [ddthetaL; ddthetaR] %Vector de aceleraciones
D = (r/(L^2))*[(M*(a^2) + 1/4 + I +(M*a*L)/r + 2*(L^2)*(2*mc + mg)),  -(M*(a^2) + 1/4 - I);
              -(M*(a^2) + 1/4 - I), (M*(a^2) + 1/4 + I -(M*a*L)/r + 2*(L^2)*(2*mc + mg))]; %Matriz de inercia
      
tau = ((r/(L^2))*[(M*(a^2) + 1/4 + I +(M*a*L)/r + 2*(L^2)*(2*mc + mg)),  -(M*(a^2) + 1/4 - I); -(M*(a^2) + 1/4 - I), (M*(a^2) + 1/4 + I -(M*a*L)/r + 2*(L^2)*(2*mc + mg))]*0)*[ddthetaL;ddthetaR]+[P/ddthetaL; P/ddthetaR];       
tau_ef = D * ddtheta;
tau_f = 0.3 * tau_ef; %Torques de friccion
tau_p = (r/2)*M*g*sin(alfa)*[1;1]; %Torques de pendiente de 30 grados
tauTot = (tau + tau_p)*1.3;
tauTot_L = tauTot(1); 
tauTot_R = tauTot(2);
